simulink model "modello"  (R2015a)
settings: Solver=ode45  StartTime=0.0  StopTime=20  RelTol=1e-3
values from neighbouring files (symbols this model uses):
  Ke = 0.0274    [parametri.m]
  Kh = 800    [parametri.m]
  L = 2.75*10^-2    (= 0.0275)    [parametri.m]
  M = 1    [parametri.m]
  R = 4    [parametri.m]
  Rd = 0.3    [parametri.m]
settings Model: Creator=dell  LastModifiedBy=dell

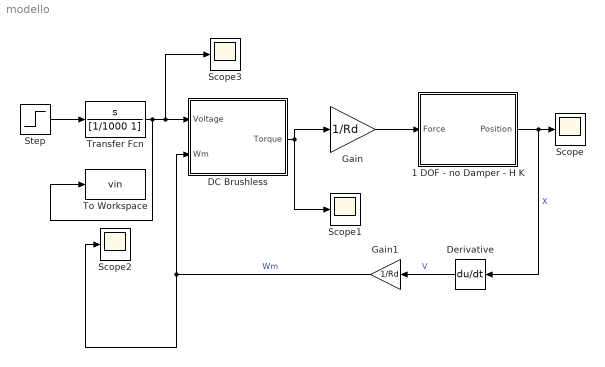
== system modello ==
  1 DOF - no Damper - H K : Subsystem
  DC Brushless : Subsystem
  Derivative : Derivative
  Gain : Gain  Gain=1/Rd
  Gain1 : Gain  Gain=1/Rd
  Scope{,1..3} (4 alike) : Scope
      Scope1 settings: YMin=-1  YMax=1
      Scope2 settings: SaveName=ScopeData3
      Scope3 settings: TimeRange=10  YMin=0  YMax=1000  SaveName=ScopeData4
  Step : Step  Time=0  SampleTime=0
  To Workspace : ToWorkspace  VariableName=vin  SaveFormat=Timeseries  SampleTime=-1
  Transfer Fcn : TransferFcn  Numerator=[1 0]  Denominator=[1/1000 1]
  wires:
  DC Brushless/1("Torque ") -> Gain/1, Scope1/1
  Gain/1 -> 1 DOF - no Damper - H K/1(Force)
  1 DOF - no Damper - H K/1(Position) -> Derivative/1, Scope/1  "X"
  Derivative/1 -> Gain1/1  "V"
  Gain1/1 -> DC Brushless/2(Wm), Scope2/1  "Wm"
  Transfer Fcn/1 -> To Workspace/1, Scope3/1, DC Brushless/1("Voltage ")
  Step/1 -> Transfer Fcn/1

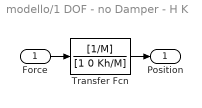
== system modello/1 DOF - no Damper - H K ==
  Force : Inport
  Transfer Fcn : TransferFcn  Numerator=[1/M]  Denominator=[1 0 Kh/M]
  Position : Outport
  wires:
  Transfer Fcn/1 -> Position/1
  Force/1 -> Transfer Fcn/1

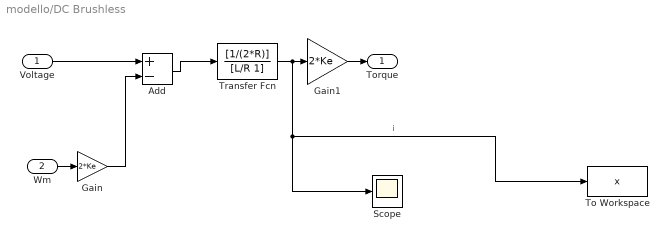
== system modello/DC Brushless ==
  "Voltage " : Inport
  Wm : Inport  Port=2
  Add : Sum  Inputs=+-
  Gain : Gain  Gain=2*Ke
  Gain1 : Gain  Gain=2*Ke
  Scope : Scope
      settings: YMin=-0.075  YMax=0.125  SaveName=ScopeData2
  To Workspace : ToWorkspace  VariableName=x  SaveFormat=Timeseries  SampleTime=-1
  Transfer Fcn : TransferFcn  Numerator=[1/(2*R)]  Denominator=[L/R 1]
  "Torque " : Outport
  wires:
  Gain1/1 -> "Torque "/1
  Transfer Fcn/1 -> To Workspace/1, Scope/1, Gain1/1  "i"
  Add/1 -> Transfer Fcn/1
  "Voltage "/1 -> Add/1
  Wm/1 -> Gain/1
  Gain/1 -> Add/2
